simulink model "verify_window_static_mdl"  (R2016b)
settings: Solver=ode45  StartTime=8*3600  StopTime=9*3600  MaxStep=600  RelTol=1e-3  EnableMultiTasking=on
libraries: carnot x4
settings Model: Creator=drhf  LastModifiedBy=drhf
settings DataIOCC: LimitDataPoints=on  SaveFormat=Array
settings OptimizationCC: DefaultParameterBehavior=Inlined  LifeSpan=inf
settings DebuggingCC: UnderspecifiedInitializationDetection=Classic  MergeDetectMultiDrivingBlocksExec=none  SolverPrmCheckMsg=warning  SFUnexpectedBacktrackingDiag=warning  SFNoUnconditionalDefaultTransitionDiag=warning  SFExecutionAtInitializationDiag=none
settings HardwareCC: ProdBitPerPointer=32  ProdBitPerSizeT=32  ProdBitPerPtrDiffT=32  ProdLargestAtomicFloat=None  ProdIntDivRoundTo=Undefined  ProdEndianess=Unspecified  ProdWordSize=32  ProdHWDeviceType=32-bit Generic
settings ModelReferenceCC: PropagateSignalLabelsOutOfModel=off
settings GRTTargetCC: TargetLangStandard=C89/C90 (ANSI)  GeneratePreprocessorConditionals=Disable all
settings ConfigComp: CovMetricSettings=dw  CovHtmlReporting=on  CovSaveCumulativeToWorkspaceVar=on  CovSaveSingleToWorkspaceVar=on  CovExternalEMLEnable=off

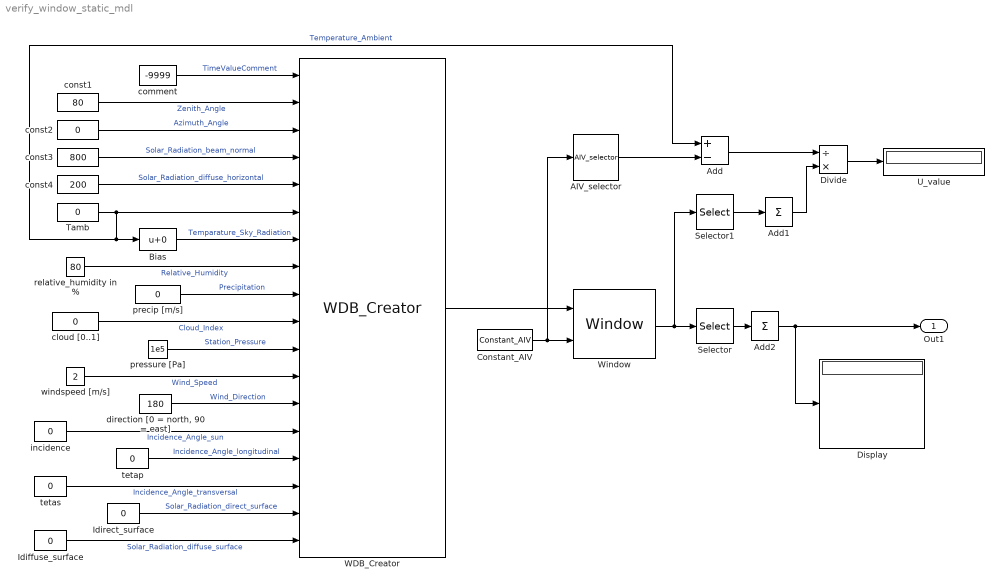
== system verify_window_static_mdl ==
  AIV_selector : carnot/Outputs/AIV_selector  e1=on  e2=off  e3=off  e4=off  e5=off  e6=off  e7=off  e8=off  e9=off
  Add : Sum  Inputs=+-
  Add1 : Sum  Inputs=1
  Add2 : Sum  Inputs=1
  Bias : Bias
  Constant_AIV : carnot/Source/Ventilation/Constant_AIV  Tsens=20  Tcon=20  Trad=20  mw=0.012  mco=0.01  rhoair=1.2  cpair=1004  pair=100000  nair=0.5
  Display : Display
  Divide : Product  Inputs=/*
  Idiffuse_surface : Constant  Value=0
  Idirect_surface : Constant  Value=0
  Selector : Selector  InputPortWidth=13  IndexOptions=Index vector (dialog)  Indices=[7 8]  OutputSizes=1
  Selector1 : Selector  InputPortWidth=13  IndexOptions=Index vector (dialog)  Indices=[7 8]  OutputSizes=1
  Tamb : Constant  Value=0
  U_value : Display
  WDB_Creator : carnot/Basic/Weather_and_Sun/WDB_Creator
  Window : carnot/Load/Houses/wall_floor/Window  windowsize=[1 1]  frame=0  pos=0  t0=20  d=[0.01 0.01]  cond=[0.5 0.5]  cwall=[.28 .28]*3600  rho=[2500 2500]  misc=[0.2 0.1 1 1]  gvalue=0.6  tau=100  dactive=[0.005 0.015]
  cloud [0..1] : Constant  Value=0
  comment : Constant  Value=-9999
  const1 : Constant  Value=80
  const2 : Constant  Value=0
  const3 : Constant  Value=800
  const4 : Constant  Value=200
  "direction [0 = north, 90 = east]" : Constant  Value=180
  incidence : Constant  Value=0
  precip [m/s] : Constant  Value=0
  pressure [Pa] : Constant  Value=1e5
  relative_humidity in % : Constant  Value=80
  tetap : Constant  Value=0
  tetas : Constant  Value=0
  windspeed [m/s] : Constant  Value=2
  Out1 : Outport
  wires:
  WDB_Creator/1 -> Window/1
  Constant_AIV/1 -> AIV_selector/1, Window/2
  Idiffuse_surface/1 -> WDB_Creator/18  "Solar_Radiation_diffuse_surface"
  Idirect_surface/1 -> WDB_Creator/17  "Solar_Radiation_direct_surface"
  tetas/1 -> WDB_Creator/16  "Incidence_Angle_transversal"
  tetap/1 -> WDB_Creator/15  "Incidence_Angle_longitudinal"
  incidence/1 -> WDB_Creator/14  "Incidence_Angle_sun"
  "direction [0 = north, 90 = east]"/1 -> WDB_Creator/13  "Wind_Direction"
  windspeed [m/s]/1 -> WDB_Creator/12  "Wind_Speed"
  pressure [Pa]/1 -> WDB_Creator/11  "Station_Pressure"
  cloud [0..1]/1 -> WDB_Creator/10  "Cloud_Index"
  precip [m/s]/1 -> WDB_Creator/9  "Precipitation"
  relative_humidity in %/1 -> WDB_Creator/8  "Relative_Humidity"
  Bias/1 -> WDB_Creator/7  "Temparature_Sky_Radiation"
  Tamb/1 -> Add/1, Bias/1, WDB_Creator/6  "Temperature_Ambient"
  const4/1 -> WDB_Creator/5  "Solar_Radiation_diffuse_horizontal"
  const2/1 -> WDB_Creator/3  "Azimuth_Angle"
  const1/1 -> WDB_Creator/2  "Zenith_Angle"
  comment/1 -> WDB_Creator/1  "TimeValueComment"
  const3/1 -> WDB_Creator/4  "Solar_Radiation_beam_normal"
  Window/1 -> Selector1/1, Selector/1
  Selector/1 -> Add2/1
  AIV_selector/1 -> Add/2
  Add/1 -> Divide/1
  Selector1/1 -> Add1/1
  Add1/1 -> Divide/2
  Divide/1 -> U_value/1
  Add2/1 -> Out1/1, Display/1
